simulink model "BitSet_TestGen6"  (R2017b)
settings: Solver=FixedStepDiscrete  StartTime=0.0  StopTime=10.0  RelTol=1e-3
undefined symbols (not defined in the file): Block_TestLib, trigger
libraries: simulink x1
settings Model: Creator=hbourbou  LastModifiedBy=hbourbou
settings DebuggingCC: ParameterOverflowMsg=none

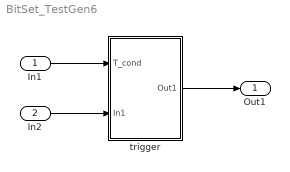
== system BitSet_TestGen6 ==
  In1 : Inport
  In2 : Inport  Port=2
  trigger : Subsystem  AncestorBlock=Block_TestLib/trigger
  Out1 : Outport
  wires:
  In1/1 -> trigger/1(T_cond)
  In2/1 -> trigger/2(In1)
  trigger/1(Out1) -> Out1/1

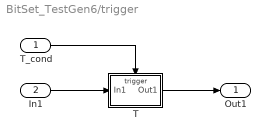
== system BitSet_TestGen6/trigger ==
  T_cond : Inport  OutDataTypeStr=boolean
  In1 : Inport  Port=2
  T : Subsystem  TreatAsAtomicUnit=on
  Out1 : Outport
  wires:
  T_cond/1 -> T/Trigger
  In1/1 -> T/1(In1)
  T/1(Out1) -> Out1/1

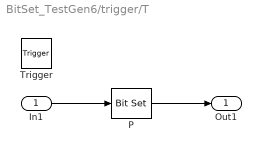
== system BitSet_TestGen6/trigger/T ==
  In1 : Inport  OutDataTypeStr=int16  PortDimensions=[1 3]
  Trigger : TriggerPort  VariantControl=Variant
  P : simulink/Logic and Bit Operations/Bit Set  iBit=0
      settings: SourceProductName=Simulink  SourceProductBaseCode=SL
  Out1 : Outport
  wires:
  In1/1 -> P/1
  P/1 -> Out1/1
